simulink model "Hauteur_Aimants_Plaque"  (R2021a)
settings: Solver=FixedStepAuto  StartTime=0.0  StopTime=10.0  RelTol=1e-3
values from neighbouring files (symbols this model uses):
  rABC = 95.20e-03    (= 0.0952)    [Constante_L.m]
settings Model: Creator=antho  LastModifiedBy=alexi

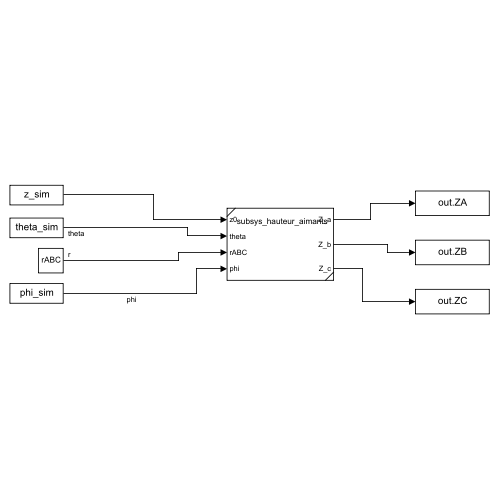
[thumbnail: Simulink's stored preview of the top-level diagram]
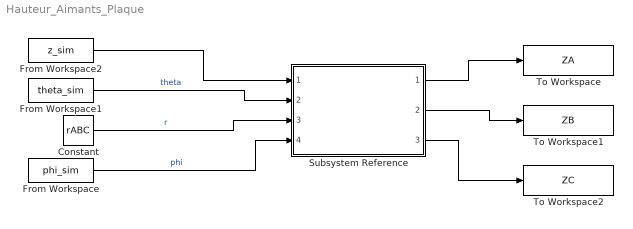
== system Hauteur_Aimants_Plaque ==
  Constant : Constant  Value=rABC
  From Workspace : FromWorkspace  VariableName=phi_sim
  From Workspace1 : FromWorkspace  VariableName=theta_sim
  From Workspace2 : FromWorkspace  VariableName=z_sim
  Subsystem Reference : Subsystem  ReferencedSubsystem=subsys_hauteur_aimants
  To Workspace : ToWorkspace  VariableName=ZA  SaveFormat=Timeseries  SampleTime=-1
  To Workspace1 : ToWorkspace  VariableName=ZB  SaveFormat=Timeseries  SampleTime=-1
  To Workspace2 : ToWorkspace  VariableName=ZC  SaveFormat=Timeseries  SampleTime=-1
  wires:
  From Workspace2/1 -> Subsystem Reference/1
  From Workspace1/1 -> Subsystem Reference/2  "theta"
  Constant/1 -> Subsystem Reference/3  "r"
  From Workspace/1 -> Subsystem Reference/4  "phi"
  Subsystem Reference/1 -> To Workspace/1
  Subsystem Reference/2 -> To Workspace1/1
  Subsystem Reference/3 -> To Workspace2/1
